simulink model "tester"  (R2014b)
settings: Solver=ode45  StartTime=0.0  StopTime=10000.0  RelTol=1e-3
settings Model: Creator=Jacek  LastModifiedBy=Jacek

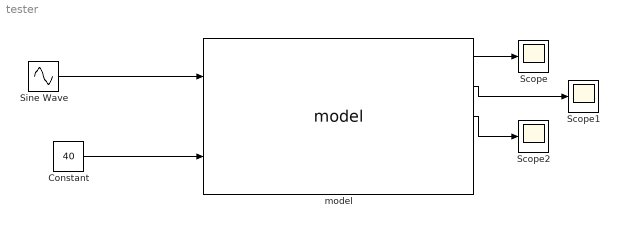
== system tester ==
  Constant : Constant  Value=40
  Scope : Scope
      settings: YMin=-1  YMax=1
  Scope1 : Scope
  Scope2 : Scope
      settings: SaveName=ScopeData2
  Sine Wave : Sin  Amplitude=10000  Frequency=0.001  Phase=1.5  SampleTime=0
  model : S-Function  FunctionName=model  EnableBusSupport=off
      mask Display: port_label('input',1,'Ein.'); port_label('input',2,'Fin.'); port_label('output',1,'Pout.'); port_label('output',2,'Tout.'); port_label('output',3,'Vout.'); port_label('output',4,'tout2.'); port_label('output',5,'DEBUG')
  wires:
  Sine Wave/1 -> model/1
  Constant/1 -> model/2
  model/1 -> Scope/1
  model/2 -> Scope1/1
  model/3 -> Scope2/1
